simulink model "top"  (Simulink 6.3)
settings: Solver=FixedStepDiscrete  StartTime=0.0  StopTime=30  FixedStep=1  RelTol=1e-3
InitFcn:
  | %% DSPBuilder Start
  | alt_dspbuilder_update_model(bdroot)
  | %% DSPBuilder End
libraries: allblocks_alteradspbuilder2 x10, simulink x1
settings Model: LastModifiedBy=delphick  StrictBusMsg=None
settings OptimizationCC: BooleanDataType=off  InlineInvariantSignals=on
settings DebuggingCC: SolverPrmCheckMsg=none
settings HardwareCC: TargetUnknown=on

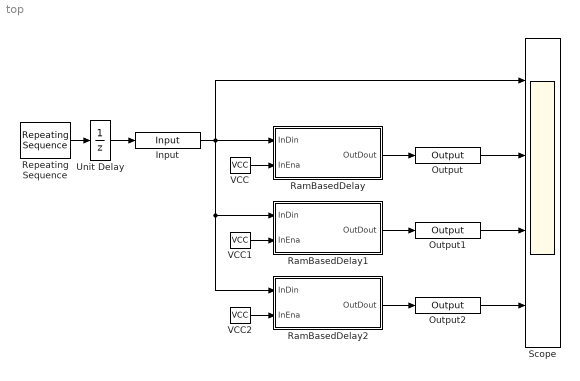
== system top ==
  Input : allblocks_alteradspbuilder2/Input  iofile=C:\workspace_clean\Documentation\DesignExamples\Tutorials\BuildingCustomLibrary\tb_top\top_Input.salt  BusType=Signed Integer  bwl=8  bwr=8  SpecifyClock=off  PORTTYPE=Input
  Output : allblocks_alteradspbuilder2/Output  iofile=C:\workspace_clean\Documentation\DesignExamples\Tutorials\BuildingCustomLibrary\tb_top\top_Output.capture  BusType=Signed Integer  bwl=8  bwr=8  PORTTYPE=Output
  Output1 : allblocks_alteradspbuilder2/Output  iofile=C:\workspace_clean\Documentation\DesignExamples\Tutorials\BuildingCustomLibrary\tb_top\top_Output1.capture  BusType=Signed Integer  bwl=8  bwr=8  PORTTYPE=Output
  Output2 : allblocks_alteradspbuilder2/Output  iofile=C:\workspace_clean\Documentation\DesignExamples\Tutorials\BuildingCustomLibrary\tb_top\top_Output2.capture  BusType=Signed Integer  bwl=8  bwr=8  PORTTYPE=Output
  RamBasedDelay : Subsystem  mask(SubSystem AlteraBlockSet){d=5}
      mask prompts: d "Delay"
      mask help:
      | RAM Based Delay Element
      |
      | Altera Corporation
      mask Display:
      | port_label('input',1,'din');
      | port_label('input',2,'ena');
      | port_label('output',1,'dout');
      | fprintf('Delay %d',d)
  RamBasedDelay1 : Subsystem  mask(SubSystem AlteraBlockSet){d=10}
      mask prompts: d "Delay"
      mask help:
      | RAM Based Delay Element
      |
      | Altera Corporation
      mask Display:
      | port_label('input',1,'din');
      | port_label('input',2,'ena');
      | port_label('output',1,'dout');
      | fprintf('Delay %d',d)
  RamBasedDelay2 : Subsystem  mask(SubSystem AlteraBlockSet){d=15}
      mask prompts: d "Delay"
      mask help:
      | RAM Based Delay Element
      |
      | Altera Corporation
      mask Display:
      | port_label('input',1,'din');
      | port_label('input',2,'ena');
      | port_label('output',1,'dout');
      | fprintf('Delay %d',d)
  Repeating Sequence : simulink/Sources/Repeating Sequence  rep_seq_t=[0 1 2 3 4 5 6 7 8]  rep_seq_y=[0 1 2 3 4 4 3 2 1]
  Scope : Scope  NumInputPorts=4
      settings: YMin=-5~-5~-5~-5  YMax=5~5~5~5
  Unit Delay : UnitDelay
  VCC : allblocks_alteradspbuilder2/VCC  SpecifyClock=off
  VCC1 : allblocks_alteradspbuilder2/VCC  SpecifyClock=off
  VCC2 : allblocks_alteradspbuilder2/VCC  SpecifyClock=off
  wires:
  Input/1 -> RamBasedDelay1/1(InDin), RamBasedDelay2/1(InDin), Scope/1, RamBasedDelay/1(InDin)
  VCC/1 -> RamBasedDelay/2(InEna)
  VCC1/1 -> RamBasedDelay1/2(InEna)
  VCC2/1 -> RamBasedDelay2/2(InEna)
  RamBasedDelay1/1(OutDout) -> Output1/1
  RamBasedDelay/1(OutDout) -> Output/1
  RamBasedDelay2/1(OutDout) -> Output2/1
  Output2/1 -> Scope/4
  Output1/1 -> Scope/3
  Output/1 -> Scope/2
  Repeating Sequence/1 -> Unit Delay/1
  Unit Delay/1 -> Input/1

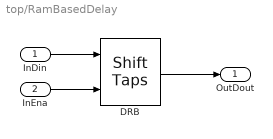
== system top/RamBasedDelay ==
  InDin : Inport
  InEna : Inport  Port=2
  DRB : allblocks_alteradspbuilder2/Shift Taps  number_of_taps=1  tap_distance=d  use_shiftout=off  use_ena=on  use_sclr=off  use_dedicated_circuitry=off  ram_type=AUTO
  OutDout : Outport
  wires:
  InDin/1 -> DRB/1
  InEna/1 -> DRB/2
  DRB/1 -> OutDout/1

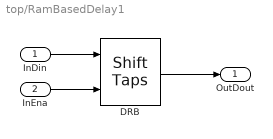
== system top/RamBasedDelay1 ==
  InDin : Inport
  InEna : Inport  Port=2
  DRB : allblocks_alteradspbuilder2/Shift Taps  number_of_taps=1  tap_distance=d  use_shiftout=off  use_ena=on  use_sclr=off  use_dedicated_circuitry=off  ram_type=AUTO
  OutDout : Outport
  wires:
  InDin/1 -> DRB/1
  InEna/1 -> DRB/2
  DRB/1 -> OutDout/1

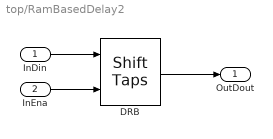
== system top/RamBasedDelay2 ==
  InDin : Inport
  InEna : Inport  Port=2
  DRB : allblocks_alteradspbuilder2/Shift Taps  number_of_taps=1  tap_distance=d  use_shiftout=off  use_ena=on  use_sclr=off  use_dedicated_circuitry=off  ram_type=AUTO
  OutDout : Outport
  wires:
  InDin/1 -> DRB/1
  InEna/1 -> DRB/2
  DRB/1 -> OutDout/1
